simulink model "sensorfn1"  (R2015a)
settings: Solver=ode45  StartTime=0.0  StopTime=10.0  RelTol=1e-3
settings Model: Creator=Ali  LastModifiedBy=Ali

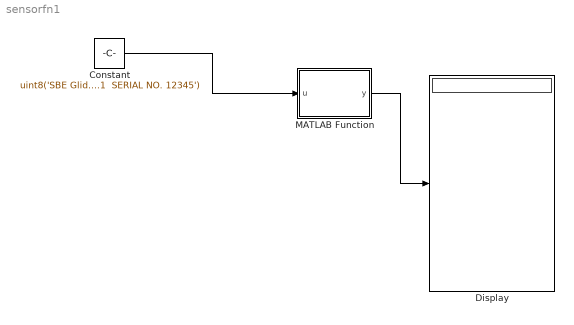
== system sensorfn1 ==
  Constant : Constant  Value="uint8('SBE Glider Payload CTD 1.2.1  SERIAL NO. 12345')"
  Display : Display
  MATLAB Function : MATLAB Function  TreatAsAtomicUnit=on
  wires:
  MATLAB Function/1(y) -> Display/1
  Constant/1 -> MATLAB Function/1(u)

== matlab function sensorfn1/MATLAB Function ==
  data: u input; y output
function y = fcn(u)
%#codegen
global bdr;
bdr=9600;
y = u;
